simulink model "shoukongFDIA"  (R2024b)
settings: Solver=FixedStepDiscrete  StartTime=0.0  StopTime=10  FixedStep=1  RelTol=1e-3
undefined symbols (not defined in the file): A, B, C, K, L, u_eq, x_eq
settings Model: Creator=54238  LastModifiedBy=54238

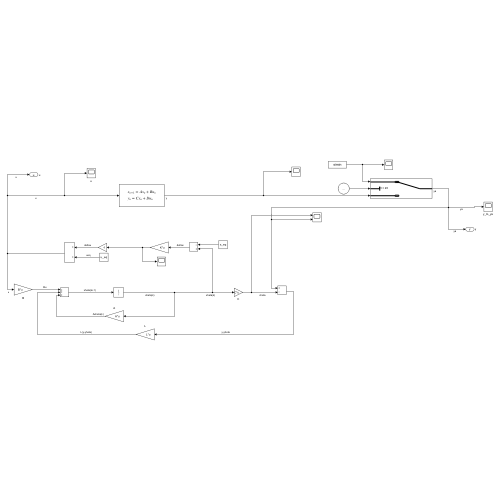
[thumbnail: Simulink's stored preview of the top-level diagram]
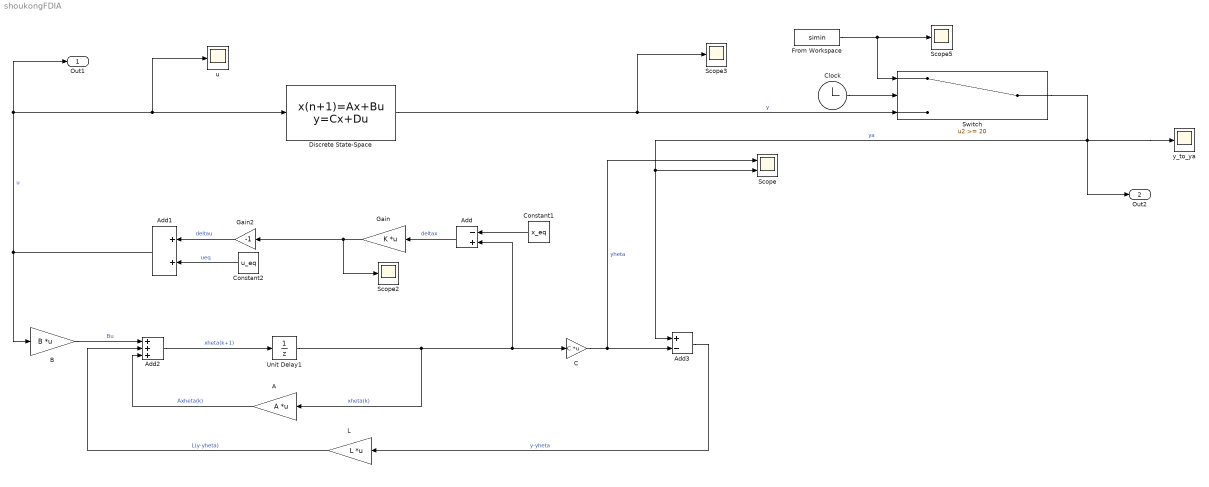
== system shoukongFDIA ==
  A : Gain  Gain=A  Multiplication=Matrix(K*u)
  Add : Sum  Inputs=-+
  Add1 : Sum
  Add2 : Sum  Inputs=+++
  Add3 : Sum  Inputs=+-
  B : Gain  Gain=B  Multiplication=Matrix(K*u)
  C : Gain  Gain=C  Multiplication=Matrix(K*u)
  Clock : Clock
  Constant1 : Constant  Value=x_eq  VectorParams1D=off
  Constant2 : Constant  Value=u_eq  VectorParams1D=off
  Discrete State-Space : DiscreteStateSpace  A=A  B=B  C=C  D=[0 0;0 0]  InitialCondition=[8 8 6 4]
  From Workspace : FromWorkspace  VariableName=simin
  Gain : Gain  Gain=K  Multiplication=Matrix(K*u)
  Gain2 : Gain  Gain=-1
  L : Gain  Gain=L  Multiplication=Matrix(K*u)
  Scope : Scope  NumInputPorts=2
  Scope2 : Scope
  Scope3 : Scope
  Scope5 : Scope
  Switch : Switch  Threshold=20  SaturateOnIntegerOverflow=off  InputSameDT=off
  Unit Delay1 : UnitDelay  SampleTime=-1  HasFrameUpgradeWarning=on
  u : Scope
  y_to_ya : Scope
  Out1 : Outport  SignalName=u  PortDimensions=[2,1]
  Out2 : Outport  Port=2  SignalName=y  PortDimensions=[2,1]
  wires:
  Unit Delay1/1 -> C/1, Add/2, A/1  "xheta(k)"
  Discrete State-Space/1 -> Scope3/1, Switch/3  "y"
  From Workspace/1 -> Scope5/1, Switch/1
  Clock/1 -> Switch/2
  Add2/1 -> Unit Delay1/1  "xheta(k+1)"
  Switch/1 -> Out2/1, Scope/2, Add3/1, y_to_ya/1  "ya"
  B/1 -> Add2/1  "Bu"
  A/1 -> Add2/3  "Axheta(k)"
  L/1 -> Add2/2  "L(y-yheta)"
  C/1 -> Scope/1, Add3/2  "yheta"
  Add/1 -> Gain/1  "deltax"
  Gain/1 -> Scope2/1, Gain2/1
  Add1/1 -> Out1/1, u/1, Discrete State-Space/1, B/1  "u"
  Gain2/1 -> Add1/1  "deltau"
  Constant1/1 -> Add/1
  Constant2/1 -> Add1/2  "ueq"
  Add3/1 -> L/1  "y-yheta"
